simulink model "EarlyReturn8_2018a"  (R2018a)
settings: Solver=FixedStepDiscrete  StartTime=0.0  StopTime=0.1  FixedStep=0.1  RelTol=1e-3  EnableMultiTasking=on
settings Model: Creator=BEAR  LastModifiedBy=bzhan
settings SolverCC: AutoInsertRateTranBlk=on
settings DataIOCC: LimitDataPoints=on
settings OptimizationCC: LifeSpan=inf
settings DebuggingCC: AllowSymbolicDim=off  SFUnexpectedBacktrackingDiag=warning  SFNoUnconditionalDefaultTransitionDiag=warning  SFExecutionAtInitializationDiag=none
settings CodeAppCC: StateflowObjectComments=on
settings GRTTargetCC: TargetLangStandard=C89/C90 (ANSI)
settings ConfigComp: CovMetricSettings=dw  CovHtmlReporting=on  CovSaveCumulativeToWorkspaceVar=on  CovSaveSingleToWorkspaceVar=on  CovShowResultsExplorer=off  CovExternalEMLEnable=off  CovSFcnEnable=off

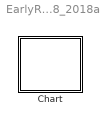
== system EarlyReturn8_2018a ==
  Chart : Stateflow chart  TreatAsAtomicUnit=on

== stateflow chart EarlyReturn8_2018a/Chart ==
  state A [parallel]
    settings: executionOrder=1
    state A1
      du: f("du_A1")
      ex: f("ex_A1")
    state A2
      en: f("en_A2")
    (default) -> A1 : {x=-1;}
    A1 -> (junction 34) [order 1] : {f("a")}
    (junction 34) -> (junction 35) : [x>0]
    (junction 35) -> A2
    A1 -> (junction 40) [order 2] : {f("c")}
    (junction 40) -> (junction 41) : E
    (junction 41) -> A2 : E
  state B [parallel]
    settings: executionOrder=2
    state B1
    state B2
      en: f("en_B2")
    state B3
      en: f("en_B3")
    (default) -> B1
    B1 -> B2 [order 2] : {f("b")}/{E;f("tb")}
    B1 -> B3 [order 1] : E
  state C [parallel]
    settings: executionOrder=3
    state C1
    state C2
      en: f("en_C2")
    state C3
      en: f("en_C3")
    C1 -> C2
    C2 -> C3
    (default) -> C1
  data: s function_input; x local
  events: E local FUNCTION_CALL_EVENT
  function f(s):
    | function f(s)
    |   fprintf(s+"\n");
